simulink model "Buckboost_COMPEL_2020_SS"  (R2019b)
settings: Solver=VariableStepAuto  StartTime=0.0  StopTime=Ts  RelTol=1e-3
undefined symbols (not defined in the file or in its folder): fixed, plecs
libraries: plecslib_extras2 x1
settings Model: Creator=jbaxte24  LastModifiedBy=jb
settings DataIOCC: ReturnWorkspaceOutputs=off
settings DebuggingCC: ArithmeticOperatorsInVariantConditions=warning
settings SFSimCC: SimUseLocalCustomCode=off  CustomCodeUndefinedFunction=UseInterfaceOnly
settings RTWCC: RTWUseLocalCustomCode=off
settings CodeAppCC: StateflowObjectComments=on

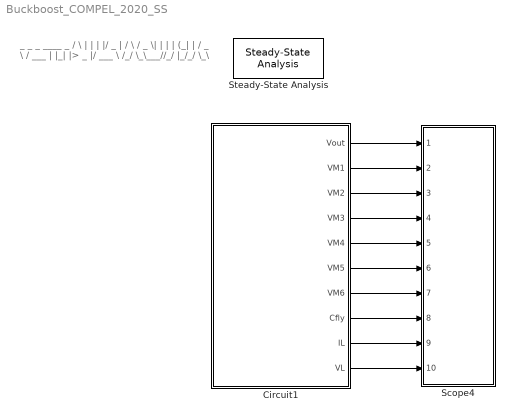
== system Buckboost_COMPEL_2020_SS ==
  note: _ _ _ ____ _
      | / \ | | | |/ _ | / \
      | / _ \| | | | (_| | / _ \
      | / ___ | |_| |> _ |/ ___ \
      | /_/ \_\___//_/ |_/_/ \_\
  Circuit1 : Subsystem  LoadFcn=plecs('sl', 200);  InitFcn=plecs('sl', 214);  StartFcn=plecs('sl', 208);  StopFcn=plecs('sl', 209);  mask(PlecsCircuit){PLECSData=<binary blob, 4092 chars, not shown>}
      mask prompts: PLECSData "PLECS Data (Do not delete or modify!)"
      mask init:
      | % PLACE CUSTOM INITIALIZATIONS ABOVE
      | % DO NOT REMOVE
      | plecs('sl', 215);
      | % DO NOT REMOVE
      settings: CopyFcn=plecs('sl', 203);  DeleteFcn=plecs('sl', 205);  UndoDeleteFcn=plecs('sl', 206);  PreSaveFcn=plecs('sl', 211);  PostSaveFcn=plecs('sl', 201);  NameChangeFcn=plecs('sl', 210);  DestroyFcn=plecs('sl', 207);  PreCopyFcn=plecs('sl', 216);  OpenFcn=plecs('sl', 202);  ErrorFcn=plerrorfcn
      mask Help: web(['file:///' fullfile(plecsdoc, 'creatingacircuit.html')])
      mask Display: disp('PLECS\nCircuit')
  Scope4 : Subsystem  LoadFcn=plecs('sl', 300);  InitFcn=plecs('sl', 314);  StartFcn=plecs('sl', 308);  StopFcn=plecs('sl', 309);  mask{Settings=<binary blob, 2300 chars, not shown>}
      mask init:
      | plecs('sl', 315);
      settings: CopyFcn=plecs('sl', 303);  DeleteFcn=plecs('sl', 305);  UndoDeleteFcn=plecs('sl', 306);  PreSaveFcn=plecs('sl', 311);  NameChangeFcn=plecs('sl', 310);  DestroyFcn=plecs('sl', 307);  OpenFcn=plecs('sl', 302);  ErrorFcn=plerrorfcn
      mask Display: plot([0.1 0.9 0.9 0.1 0.1], [0.9 0.9 0.5 0.5 0.9])
  Steady-State Analysis : plecslib_extras2/Analysis Tools/Steady-State Analysis  Period=fixed  TriggerType=rising  TimeSpan=1e-06  TStart=0  MaxIter=10000  Tolerance=1e-5  Display=iteration  HideScopes=off  HiddenStates=error  FinalStateName=xSteadyState  NCycles=3  JPert=1e-4  JacobianCalculation=fast  NInitCycles=0
      settings: SourceProductName=PLECS Extras
  wires:
  Circuit1/9(IL) -> Scope4/9(9)
  Circuit1/5(VM4) -> Scope4/5(5)
  Circuit1/3(VM2) -> Scope4/3(3)
  Circuit1/7(VM6) -> Scope4/7(7)
  Circuit1/2(VM1) -> Scope4/2(2)
  Circuit1/8(Cfly) -> Scope4/8(8)
  Circuit1/4(VM3) -> Scope4/4(4)
  Circuit1/10(VL) -> Scope4/10(10)
  Circuit1/1(Vout) -> Scope4/1(1)
  Circuit1/6(VM5) -> Scope4/6(6)

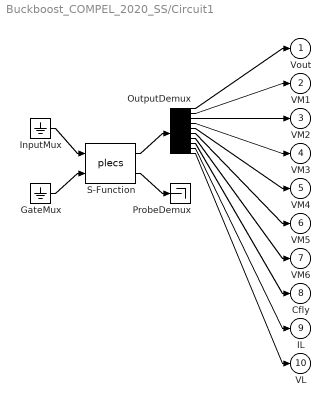
== system Buckboost_COMPEL_2020_SS/Circuit1 ==
  " GateMux " : Ground
  " InputMux " : Ground
  " OutputDemux " : Demux  Outputs=[ 1 1 1 1 1 1 1 1 1 1 ]
  " ProbeDemux " : Terminator
  " S-Function " : S-Function  FunctionName=plecs  SFunctionDeploymentMode=off  EnableBusSupport=off
  Vout : Outport  PortDimensions=1
  VM1 : Outport  Port=2  PortDimensions=1
  VM2 : Outport  Port=3  PortDimensions=1
  VM3 : Outport  Port=4  PortDimensions=1
  VM4 : Outport  Port=5  PortDimensions=1
  VM5 : Outport  Port=6  PortDimensions=1
  VM6 : Outport  Port=7  PortDimensions=1
  Cfly : Outport  Port=8  PortDimensions=1
  IL : Outport  Port=9  PortDimensions=1
  VL : Outport  Port=10  PortDimensions=1
  wires:
  " InputMux "/1 -> " S-Function "/1
  " GateMux "/1 -> " S-Function "/2
  " S-Function "/1 -> " OutputDemux "/1
  " S-Function "/2 -> " ProbeDemux "/1
  " OutputDemux "/1 -> Vout/1
  " OutputDemux "/2 -> VM1/1
  " OutputDemux "/3 -> VM2/1
  " OutputDemux "/4 -> VM3/1
  " OutputDemux "/5 -> VM4/1
  " OutputDemux "/6 -> VM5/1
  " OutputDemux "/7 -> VM6/1
  " OutputDemux "/8 -> Cfly/1
  " OutputDemux "/9 -> IL/1
  " OutputDemux "/10 -> VL/1

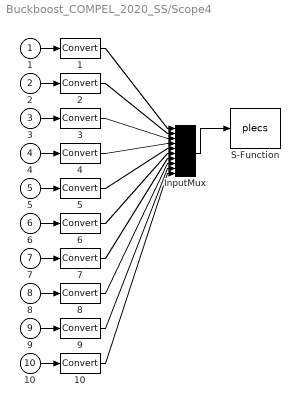
== system Buckboost_COMPEL_2020_SS/Scope4 ==
  1 : Inport
  2 : Inport  Port=2
  3 : Inport  Port=3
  4 : Inport  Port=4
  5 : Inport  Port=5
  6 : Inport  Port=6
  7 : Inport  Port=7
  8 : Inport  Port=8
  9 : Inport  Port=9
  10 : Inport  Port=10
  " 1 " : DataTypeConversion  SaturateOnIntegerOverflow=on  RndMeth=Zero
  " 10 " : DataTypeConversion  SaturateOnIntegerOverflow=on  RndMeth=Zero
  " 2 " : DataTypeConversion  SaturateOnIntegerOverflow=on  RndMeth=Zero
  " 3 " : DataTypeConversion  SaturateOnIntegerOverflow=on  RndMeth=Zero
  " 4 " : DataTypeConversion  SaturateOnIntegerOverflow=on  RndMeth=Zero
  " 5 " : DataTypeConversion  SaturateOnIntegerOverflow=on  RndMeth=Zero
  " 6 " : DataTypeConversion  SaturateOnIntegerOverflow=on  RndMeth=Zero
  " 7 " : DataTypeConversion  SaturateOnIntegerOverflow=on  RndMeth=Zero
  " 8 " : DataTypeConversion  SaturateOnIntegerOverflow=on  RndMeth=Zero
  " 9 " : DataTypeConversion  SaturateOnIntegerOverflow=on  RndMeth=Zero
  " InputMux " : Mux  Inputs=10
  " S-Function " : S-Function  FunctionName=plecs  SFunctionDeploymentMode=off  EnableBusSupport=off
  wires:
  " InputMux "/1 -> " S-Function "/1
  1/1 -> " 1 "/1
  " 1 "/1 -> " InputMux "/1
  2/1 -> " 2 "/1
  " 2 "/1 -> " InputMux "/2
  3/1 -> " 3 "/1
  " 3 "/1 -> " InputMux "/3
  4/1 -> " 4 "/1
  " 4 "/1 -> " InputMux "/4
  5/1 -> " 5 "/1
  " 5 "/1 -> " InputMux "/5
  6/1 -> " 6 "/1
  " 6 "/1 -> " InputMux "/6
  7/1 -> " 7 "/1
  " 7 "/1 -> " InputMux "/7
  8/1 -> " 8 "/1
  " 8 "/1 -> " InputMux "/8
  9/1 -> " 9 "/1
  " 9 "/1 -> " InputMux "/9
  10/1 -> " 10 "/1
  " 10 "/1 -> " InputMux "/10
